simulink model "MatLab5"  (Simulink 8.3)
settings: Solver=ode45  StartTime=0.0  StopTime=100  MaxStep=0.01  RelTol=1e-3
values from neighbouring files (symbols this model uses):
  A = [0 1  0              0 ... (first row only)    [MatLab4p.m]    (also in MatLab5p.m = [     0        1       0        0; MatLab6p_solucao4.m = [     0        1       0        0; MatLab7p.m = [0 1; -5*sqrt(2) -1]; pplane8.m = [)
  Am = blkdiag(M,M)    [MatLab5p.m]    (also in MatLab6p_solucao4.m; questao2Miguel.m = blkdiag(M); questao2MiguelFinal.m = blkdiag(M))
  B = [0; 1/M; 0; -1/(M*L)]    [MatLab4p.m]    (also in MatLab5p.m = [ 0    0; MatLab6p_solucao4.m = [ 0    0; MatLab7p.m = [0 ; 10]; pplane8.m = real(A))
  Bm = blkdiag(N,N)    [MatLab5p.m]    (also in MatLab6p_solucao4.m; questao2Miguel.m = blkdiag(N); questao2MiguelFinal.m = blkdiag(N))
  C = [1 0 0 0]    [MatLab4p.m]    (also in MatLab5p.m = [1 0 0 0; MatLab6p_solucao4.m = [1 0 0 0; MatLab7p.m = [1 0]; pplane8.m = imag(A))
  Dsim = zeros(4,1)    [MatLab4p.m]    (also in MatLab5p.m = zeros(4,2); MatLab6p_solucao4.m = zeros(4,2); questao2Miguel.m; questao2MiguelFinal.m)
  K = place(A,B,[-3 -3.05 -3.1 -3.15])    [MatLab4p.m]    (also in MatLab5p.m = Ka(:,1:4); MatLab6p_solucao4.m = Ka(:,1:4); MatLab7p.m = place(A,B,[-4 -4.05]); pplane8.m = kk +2*(jj-1))
  Km = Ka(:,5:10)    [MatLab5p.m]    (also in MatLab6p_solucao4.m = Ka(:,5:12); MatLab7p.m = Ka(1,3); questao2Miguel.m = Ka(5); questao2MiguelFinal.m = Ka(5))
  x0 = [0 0 pi/4 0]    [MatLab4p.m]    (also in MatLab5p.m = [1 0.5 1 0.1]; MatLab6p_solucao4.m = [0 0 0 0]; MatLab7p.m = [0 ; 0]; questao2Miguel.m = [0 0.01 0.3 0])
settings Model: Creator=hector  LastModifiedBy=hector
settings DataIOCC: SignalLoggingSaveFormat=Dataset
settings DebuggingCC: UnderspecifiedInitializationDetection=Simplified  StateNameClashWarn=none
settings GRTTargetCC: CombineOutputUpdateFcns=on  GRTInterface=off

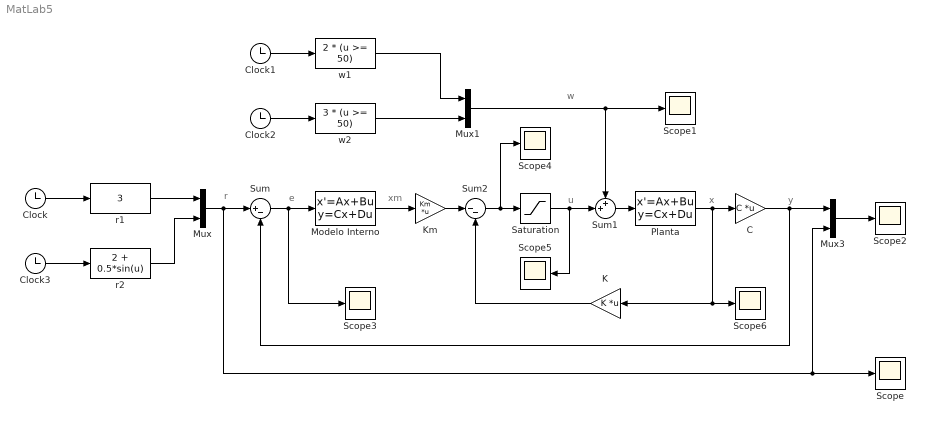
== system MatLab5 ==
  note: w
  note: u
  note: xm
  note: e
  note: r
  note: x
  note: y
  C : Gain  Gain=C  Multiplication=Matrix(K*u)
  Clock{,1..3} (4 alike) : Clock
  K : Gain  Gain=K  Multiplication=Matrix(K*u)
  Km : Gain  Gain=Km  Multiplication=Matrix(K*u)
  Modelo Interno : StateSpace  A=Am  B=Bm  C=eye(6)  D=zeros(6,2)  X0=zeros(6,1)
  Mux : Mux  Inputs=2
  Mux1 : Mux  Inputs=2
  Mux3 : Mux  Inputs=2
  Planta : StateSpace  A=A  B=B  C=eye(4)  D=Dsim  X0=x0
  Saturation : Saturate  UpperLimit=20  LowerLimit=-20
  Scope{,1..6} (7 alike) : Scope
      Scope2 settings: YMin=1.9  YMax=3.3  SaveName=ScopeData2
      Scope3 settings: YMin=-0.035  YMax=0.0025  SaveName=ScopeData3
      Scope4 settings: YMin=-2.5  YMax=50  SaveName=ScopeData4
      Scope5 settings: YMin=1  YMax=6  SaveName=ScopeData5
      Scope6 settings: ShowLegends=on  YMin=-0.5  YMax=3.25  SaveName=ScopeData6
  Sum : Sum  Inputs=|+-
  Sum1 : Sum  Inputs=++|
  Sum2 : Sum  Inputs=|--
  r1 : Fcn  Expr=3
  r2 : Fcn  Expr=2 + 0.5*sin(u)
  w1 : Fcn  Expr=2 * (u >= 50)
  w2 : Fcn  Expr=3 * (u >= 50)
  wires:
  Clock1/1 -> w1/1
  Sum/1 -> Modelo Interno/1, Scope3/1
  Sum1/1 -> Planta/1
  Clock2/1 -> w2/1
  r1/1 -> Mux/1
  Clock/1 -> r1/1
  Clock3/1 -> r2/1
  r2/1 -> Mux/2
  w1/1 -> Mux1/1
  w2/1 -> Mux1/2
  Mux1/1 -> Sum1/1, Scope1/1
  Planta/1 -> C/1, Scope6/1, K/1
  Mux3/1 -> Scope2/1
  Sum2/1 -> Saturation/1, Scope4/1
  Km/1 -> Sum2/1
  Modelo Interno/1 -> Km/1
  K/1 -> Sum2/2
  C/1 -> Mux3/1, Sum/2
  Mux/1 -> Sum/1, Scope/1, Mux3/2
  Saturation/1 -> Sum1/2, Scope5/1
